simulink model "close_loop_system_retour_etat_int_cor"  (Simulink 7.7)
settings: Solver=ode45  StartTime=0.0  StopTime=10.0  RelTol=1e-3
values from neighbouring files (symbols this model uses):
  Jt = 0.002    [BE7_trame.m]
  K_int = place(sys_int.a, sys_int.b(:,1), Po)    [BE7_trame.m]
  K_stat_int = MK_stat_int(1,1)    [BE7_trame.m]
  Kci = 1    [BE7_trame.m]
  Kcp = 1    [BE7_trame.m]
  Kcv = 0.0314    [BE7_trame.m]
  Ke = 0.2    [BE7_trame.m]
  Kg = 0.2    [BE7_trame.m]
  Le = 0.002    [BE7_trame.m]
  N = 300    [BE7_trame.m]
  Re = 2    [BE7_trame.m]
  sys_int = linmod('open_loop_system_retour_etat_int')    [BE7_trame.m]
libraries: simulink x2
settings Model: Creator=Anthony  LastModifiedBy=Anthony

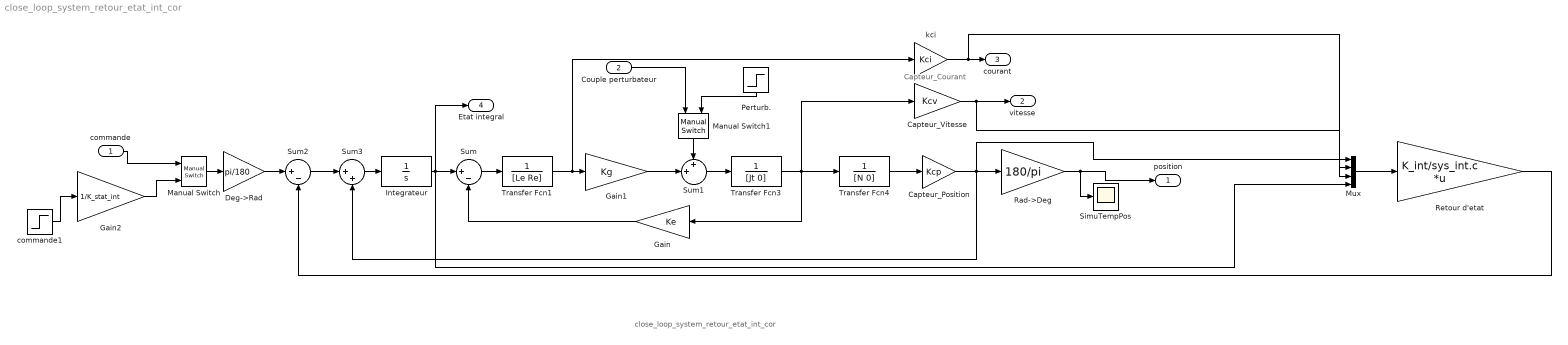
== system close_loop_system_retour_etat_int_cor ==
  note: close_loop_system_retour_etat_int_cor
  note: Capteur_Courant
  commande : Inport
  Couple perturbateur : Inport  Port=2
  Capteur_Position : Gain  Gain=Kcp  SaturateOnIntegerOverflow=on  OutDataTypeStr=Inherit: Same as input  ParamDataTypeStr=Inherit: Same as input
  Capteur_Vitesse : Gain  Gain=Kcv  SaturateOnIntegerOverflow=on  OutDataTypeStr=Inherit: Same as input  ParamDataTypeStr=Inherit: Same as input
  Deg->Rad : Gain  Gain=pi/180
  Gain : Gain  Gain=Ke  SaturateOnIntegerOverflow=on  OutDataTypeStr=Inherit: Same as input  ParamDataTypeStr=Inherit: Same as input
  Gain1 : Gain  Gain=Kg  SaturateOnIntegerOverflow=on  OutDataTypeStr=Inherit: Same as input  ParamDataTypeStr=Inherit: Same as input
  Gain2 : Gain  Gain=1/K_stat_int
  Integrateur : TransferFcn  Denominator=[1 0]
  Manual Switch : simulink/Signal Routing/Manual Switch  SystemSampleTime=-1  sw=0  action=0  varsize=off
  Manual Switch1 : simulink/Signal Routing/Manual Switch  SystemSampleTime=-1  sw=0  action=0  varsize=off
  Mux : Mux
  Perturb. : Step  Time=5  After=5  SampleTime=0
  Rad->Deg : Gain  Gain=180/pi
  Retour d'etat : Gain  Gain=K_int/sys_int.c  Multiplication=Matrix(K*u)
  SimuTempPos : Scope
      settings: TimeRange=0.3783783783783781  YMin=65.46786922209697  YMax=68.78241262683201
  Sum : Sum  Inputs=|+-  SaturateOnIntegerOverflow=on  InputSameDT=on  OutDataTypeStr=Inherit: Same as first input
  Sum1 : Sum  Inputs=++|  SaturateOnIntegerOverflow=on  InputSameDT=on  OutDataTypeStr=Inherit: Same as first input
  Sum2 : Sum  Inputs=|+-
  Sum3 : Sum  Inputs=|++
  Transfer Fcn1 : TransferFcn  Denominator=[Le Re]
  Transfer Fcn3 : TransferFcn  Denominator=[Jt 0]
  Transfer Fcn4 : TransferFcn  Denominator=[N 0]
  commande1 : Step  Time=0  After=100  SampleTime=0
  kci : Gain  Gain=Kci  SaturateOnIntegerOverflow=on  OutDataTypeStr=Inherit: Same as input  ParamDataTypeStr=Inherit: Same as input
  position : Outport
  vitesse : Outport  Port=2
  courant : Outport  Port=3
  Etat integral : Outport  Port=4
  wires:
  Sum/1 -> Transfer Fcn1/1
  Transfer Fcn1/1 -> Gain1/1, kci/1
  Transfer Fcn3/1 -> Capteur_Vitesse/1, Transfer Fcn4/1, Gain/1
  Gain/1 -> Sum/2
  Transfer Fcn4/1 -> Capteur_Position/1
  Gain1/1 -> Sum1/2
  Sum1/1 -> Transfer Fcn3/1
  commande/1 -> Manual Switch/1
  Couple perturbateur/1 -> Manual Switch1/1
  Manual Switch1/1 -> Sum1/1
  kci/1 -> courant/1, Mux/3
  Mux/1 -> Retour d'etat/1
  Capteur_Vitesse/1 -> vitesse/1, Mux/2
  Retour d'etat/1 -> Sum2/2
  Sum2/1 -> Sum3/1
  Integrateur/1 -> Sum/1, Etat integral/1, Mux/4
  Sum3/1 -> Integrateur/1
  Deg->Rad/1 -> Sum2/1
  Manual Switch/1 -> Deg->Rad/1
  Rad->Deg/1 -> position/1, SimuTempPos/1
  Capteur_Position/1 -> Rad->Deg/1, Mux/1, Sum3/2
  Gain2/1 -> Manual Switch/2
  commande1/1 -> Gain2/1
  Perturb./1 -> Manual Switch1/2
